simulink model "GAIN5"  (R2013a)
settings: Solver=ode45  StartTime=0.0  StopTime=10.0  RelTol=1e-3
settings Model: Creator=tibbs2010  LastModifiedBy=tibbs2010

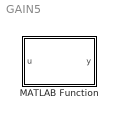
== system GAIN5 ==
  MATLAB Function : MATLAB Function  TreatAsAtomicUnit=on

== matlab function GAIN5/MATLAB Function ==
  data: u input; y output
function y = fcn(u)
%#codegen

y = u*5;
